simulink model "threebFMSquareWave"  (R2018a)
settings: Solver=VariableStepAuto  StartTime=0.0  StopTime=1  RelTol=1e-3
libraries: commanabbnd3 x2
settings Model: Creator=Neo  LastModifiedBy=Neo

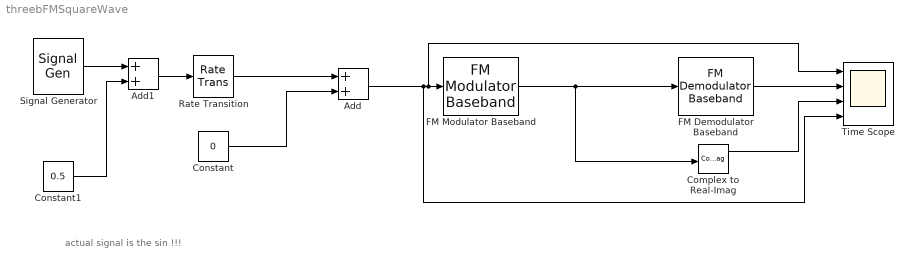
== system threebFMSquareWave ==
  note: actual signal is the sin !!!
  Add : Sum
  Add1 : Sum
  Complex to Real-Imag : ComplexToRealImag
  Constant : Constant  Value=0
  Constant1 : Constant  Value=0.5
  "FM Demodulator Baseband " : commanabbnd3/FM Demodulator Baseband   FrequencyDeviation=100  SimulateUsing=Code generation
      settings: SourceProductName=Communications System Toolbox  SourceProductBaseCode=CM
  FM Modulator Baseband : commanabbnd3/FM Modulator Baseband  FrequencyDeviation=100  SimulateUsing=Code generation
      settings: SourceProductName=Communications System Toolbox  SourceProductBaseCode=CM
  Rate Transition : RateTransition  OutPortSampleTime=0.00001
  Signal Generator : SignalGenerator  WaveForm=sawtooth  Amplitude=0.5  Frequency=5
  Time Scope : Scope  NumInputPorts=4
  wires:
  Rate Transition/1 -> Add/1
  FM Modulator Baseband/1 -> "FM Demodulator Baseband "/1, Complex to Real-Imag/1
  Add/1 -> Time Scope/4, Time Scope/1, FM Modulator Baseband/1
  Constant/1 -> Add/2
  Complex to Real-Imag/1 -> Time Scope/3
  "FM Demodulator Baseband "/1 -> Time Scope/2
  Add1/1 -> Rate Transition/1
  Signal Generator/1 -> Add1/1
  Constant1/1 -> Add1/2
